simulink model "standModel"  (R2020b)
settings: Solver=VariableStepAuto  StartTime=0.0  StopTime=10.0  RelTol=1e-3
model workspace: external: MAT-File C:\Code\KillerWhaleSim\standParams.mat (data not in the file)
undefined symbols (not defined in the file or in its folder): standParams, X, Y, Z
libraries: sm_lib x713, nesl_utility x1
(part 1 of 11)
settings Model: Creator=roadrunner  LastModifiedBy=roadrunner

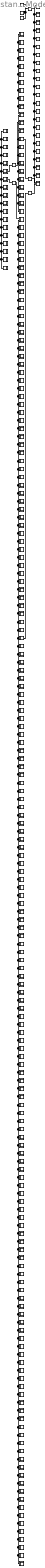
== system standModel ==
  Bracket_16_RIGID : Subsystem
  Bracket_17_RIGID : Subsystem
  Bracket_18_RIGID : Subsystem
  Bracket_19_RIGID : Subsystem
  Bracket_20_RIGID : Subsystem
  Bracket_21_RIGID : Subsystem
  Frame_Part_5_RIGID : Subsystem
  Frame_Part_6_RIGID : Subsystem
  Hinge_10_RIGID : Subsystem
  Hinge_11_RIGID : Subsystem
  Lock_tabs_13_RIGID : Subsystem
  Lock_tabs_15_RIGID : Subsystem
  Lock_tabs_16_RIGID : Subsystem
  Lock_tabs_18_RIGID : Subsystem
  MechanismConfiguration : sm_lib/Utilities/Mechanism Configuration  UniformGravity=Constant  GravityVector=[0 -9.80665 0]  GravityVectorUnits=m/s^2  GravityUnits=m/s^2  LinearizationDelta=0.001  JointModeTransitionNonlinearIterations=2
  Part_132_2_RIGID : Subsystem
  Part_133_2_RIGID : Subsystem
  Part_144_1_RIGID : Subsystem
  Part_145_1_RIGID : Subsystem
  Part_146_1_RIGID : Subsystem
  Part_147_1_RIGID : Subsystem
  Part_148_1_RIGID : Subsystem
  Part_149_1_RIGID : Subsystem
  Part_150_1_RIGID : Subsystem
  Part_151_1_RIGID : Subsystem
  Part_152_1_RIGID : Subsystem
  Part_153_1_RIGID : Subsystem
  Part_154_1_RIGID : Subsystem
  Part_155_1_RIGID : Subsystem
  Part_156_2_RIGID : Subsystem
  Part_157_2_RIGID : Subsystem
  Part_168_1_RIGID : Subsystem
  Part_169_1_RIGID : Subsystem
  Part_170_1_RIGID : Subsystem
  Part_171_1_RIGID : Subsystem
  Part_172_1_RIGID : Subsystem
  Part_173_1_RIGID : Subsystem
  Part_174_1_RIGID : Subsystem
  Part_175_1_RIGID : Subsystem
  Part_176_1_RIGID : Subsystem
  Part_177_1_RIGID : Subsystem
  Part_178_1_RIGID : Subsystem
  Part_179_1_RIGID : Subsystem
  Part_186_1_RIGID : Subsystem
  Part_187_1_RIGID : Subsystem
  Part_188_1_RIGID : Subsystem
  Part_190_1_RIGID : Subsystem
  Part_191_1_RIGID : Subsystem
  Part_192_1_RIGID : Subsystem
  Part_193_1_RIGID : Subsystem
  Part_194_1_RIGID : Subsystem
  Part_195_1_RIGID : Subsystem
  Part_196_1_RIGID : Subsystem
  Part_197_1_RIGID : Subsystem
  Part_198_2_RIGID : Subsystem
  Part_199_2_RIGID : Subsystem
  Part_200_2_RIGID : Subsystem
  Part_204_2_RIGID : Subsystem
  Part_205_2_RIGID : Subsystem
  Part_206_2_RIGID : Subsystem
  Part_213_1_RIGID : Subsystem
  Part_289_1_RIGID : Subsystem
  Part_318_1_RIGID : Subsystem
  Part_319_1_RIGID : Subsystem
  Part_322_1_RIGID : Subsystem
  Part_325_1_RIGID : Subsystem
  Part_328_1_RIGID : Subsystem
  Part_331_1_RIGID : Subsystem
  Part_334_1_RIGID : Subsystem
  Part_337_1_RIGID : Subsystem
  Part_340_1_RIGID : Subsystem
  Part_343_1_RIGID : Subsystem
  Part_346_1_RIGID : Subsystem
  Part_349_1_RIGID : Subsystem
  Part_350_2_RIGID : Subsystem
  Part_351_2_RIGID : Subsystem
  Part_352_2_RIGID : Subsystem
  Part_353_2_RIGID : Subsystem
  Part_355_2_RIGID : Subsystem
  Part_356_2_RIGID : Subsystem
  Part_357_2_RIGID : Subsystem
  Part_358_2_RIGID : Subsystem
  Part_359_2_RIGID : Subsystem
  Part_360_1_RIGID : Subsystem
  Part_361_1_RIGID : Subsystem
  Part_362_1_RIGID : Subsystem
  Part_363_1_RIGID : Subsystem
  Part_364_1_RIGID : Subsystem
  Part_365_1_RIGID : Subsystem
  Part_366_1_RIGID : Subsystem
  Part_367_1_RIGID : Subsystem
  Part_368_1_RIGID : Subsystem
  Part_369_1_RIGID : Subsystem
  Part_370_1_RIGID : Subsystem
  Part_371_1_RIGID : Subsystem
  Part_372_1_RIGID : Subsystem
  Part_373_1_RIGID : Subsystem
  Part_374_1_RIGID : Subsystem
  Part_375_1_RIGID : Subsystem
  Part_380_1_RIGID : Subsystem
  Part_386_1_RIGID : Subsystem
  Part_387_1_RIGID : Subsystem
  Part_393_1_RIGID : Subsystem
  Part_399_1_RIGID : Subsystem
  Part_400_1_RIGID : Subsystem
  Part_406_1_RIGID : Subsystem
  Part_412_1_RIGID : Subsystem
  Part_413_1_RIGID : Subsystem
  Revolute1 : sm_lib/Joints/Revolute Joint  JointMode=Normal  SenseConstraintForce=off  SenseConstraintForceX=off  SenseConstraintForceY=off  SenseConstraintForceZ=off  SenseConstraintTorque=off  SenseConstraintTorqueX=off  SenseConstraintTorqueY=off  SenseConstraintTorqueZ=off  SenseTotalForce=off  SenseTotalForceX=off  SenseTotalForceY=off  SenseTotalForceZ=off  SenseTotalTorque=off  SenseTotalTorqueX=off  SenseTotalTorqueY=off  SenseTotalTorqueZ=off  CompositeWrenchDir=FollowerOnBase  CompositeWrenchFrame=BaseFrame  EquilibriumPosition=0  EquilibriumPositionUnits=deg  SpringStiffness=0  SpringStiffnessUnits=N*m/deg  DampingCoefficient=0  DampingCoefficientUnits=N*m/(deg/s)  TorqueActuationMode=NoTorque  MotionActuationMode=ComputedMotion  SensePosition=off  SenseVelocity=off  SenseAcceleration=off  SenseTorqueForce=off  SenseLowerLimitTorqueForce=off  SenseUpperLimitTorqueForce=off  LowerLimitSpecify=off  LowerLimitBound=-90  LowerLimitBoundUnits=deg  LowerLimitStiffness=1e4  LowerLimitStiffnessUnits=N*m/deg  LowerLimitDamping=10  LowerLimitDampingUnits=N*m/(deg/s)  LowerLimitTransitionRegionWidth=0.1  LowerLimitTransitionRegionWidthUnits=deg  UpperLimitSpecify=off  UpperLimitBound=90  UpperLimitBoundUnits=deg  UpperLimitStiffness=1e4  UpperLimitStiffnessUnits=N*m/deg  UpperLimitDamping=10  UpperLimitDampingUnits=N*m/(deg/s)  UpperLimitTransitionRegionWidth=0.1  UpperLimitTransitionRegionWidthUnits=deg  PositionTargetSpecify=on  PositionTargetPriority=Low  PositionTargetValue=standParams.RevoluteJoint(1).Rz.Pos  PositionTargetValueUnits=deg  VelocityTargetSpecify=off  VelocityTargetPriority=High  VelocityTargetValue=0  VelocityTargetValueUnits=deg/s
  Revolute2 : sm_lib/Joints/Revolute Joint  JointMode=Normal  SenseConstraintForce=off  SenseConstraintForceX=off  SenseConstraintForceY=off  SenseConstraintForceZ=off  SenseConstraintTorque=off  SenseConstraintTorqueX=off  SenseConstraintTorqueY=off  SenseConstraintTorqueZ=off  SenseTotalForce=off  SenseTotalForceX=off  SenseTotalForceY=off  SenseTotalForceZ=off  SenseTotalTorque=off  SenseTotalTorqueX=off  SenseTotalTorqueY=off  SenseTotalTorqueZ=off  CompositeWrenchDir=FollowerOnBase  CompositeWrenchFrame=BaseFrame  EquilibriumPosition=0  EquilibriumPositionUnits=deg  SpringStiffness=0  SpringStiffnessUnits=N*m/deg  DampingCoefficient=0  DampingCoefficientUnits=N*m/(deg/s)  TorqueActuationMode=NoTorque  MotionActuationMode=ComputedMotion  SensePosition=off  SenseVelocity=off  SenseAcceleration=off  SenseTorqueForce=off  SenseLowerLimitTorqueForce=off  SenseUpperLimitTorqueForce=off  LowerLimitSpecify=off  LowerLimitBound=-90  LowerLimitBoundUnits=deg  LowerLimitStiffness=1e4  LowerLimitStiffnessUnits=N*m/deg  LowerLimitDamping=10  LowerLimitDampingUnits=N*m/(deg/s)  LowerLimitTransitionRegionWidth=0.1  LowerLimitTransitionRegionWidthUnits=deg  UpperLimitSpecify=off  UpperLimitBound=90  UpperLimitBoundUnits=deg  UpperLimitStiffness=1e4  UpperLimitStiffnessUnits=N*m/deg  UpperLimitDamping=10  UpperLimitDampingUnits=N*m/(deg/s)  UpperLimitTransitionRegionWidth=0.1  UpperLimitTransitionRegionWidthUnits=deg  PositionTargetSpecify=off  PositionTargetPriority=High  PositionTargetValue=0  PositionTargetValueUnits=deg  VelocityTargetSpecify=off  VelocityTargetPriority=High  VelocityTargetValue=0  VelocityTargetValueUnits=deg/s
  Revolute3 : sm_lib/Joints/Revolute Joint  JointMode=Normal  SenseConstraintForce=off  SenseConstraintForceX=off  SenseConstraintForceY=off  SenseConstraintForceZ=off  SenseConstraintTorque=off  SenseConstraintTorqueX=off  SenseConstraintTorqueY=off  SenseConstraintTorqueZ=off  SenseTotalForce=off  SenseTotalForceX=off  SenseTotalForceY=off  SenseTotalForceZ=off  SenseTotalTorque=off  SenseTotalTorqueX=off  SenseTotalTorqueY=off  SenseTotalTorqueZ=off  CompositeWrenchDir=FollowerOnBase  CompositeWrenchFrame=BaseFrame  EquilibriumPosition=0  EquilibriumPositionUnits=deg  SpringStiffness=0  SpringStiffnessUnits=N*m/deg  DampingCoefficient=0  DampingCoefficientUnits=N*m/(deg/s)  TorqueActuationMode=NoTorque  MotionActuationMode=ComputedMotion  SensePosition=off  SenseVelocity=off  SenseAcceleration=off  SenseTorqueForce=off  SenseLowerLimitTorqueForce=off  SenseUpperLimitTorqueForce=off  LowerLimitSpecify=off  LowerLimitBound=-90  LowerLimitBoundUnits=deg  LowerLimitStiffness=1e4  LowerLimitStiffnessUnits=N*m/deg  LowerLimitDamping=10  LowerLimitDampingUnits=N*m/(deg/s)  LowerLimitTransitionRegionWidth=0.1  LowerLimitTransitionRegionWidthUnits=deg  UpperLimitSpecify=off  UpperLimitBound=90  UpperLimitBoundUnits=deg  UpperLimitStiffness=1e4  UpperLimitStiffnessUnits=N*m/deg  UpperLimitDamping=10  UpperLimitDampingUnits=N*m/(deg/s)  UpperLimitTransitionRegionWidth=0.1  UpperLimitTransitionRegionWidthUnits=deg  PositionTargetSpecify=on  PositionTargetPriority=Low  PositionTargetValue=standParams.RevoluteJoint(2).Rz.Pos  PositionTargetValueUnits=deg  VelocityTargetSpecify=off  VelocityTargetPriority=High  VelocityTargetValue=0  VelocityTargetValueUnits=deg/s
  Revolute4 : sm_lib/Joints/Revolute Joint  JointMode=Normal  SenseConstraintForce=off  SenseConstraintForceX=off  SenseConstraintForceY=off  SenseConstraintForceZ=off  SenseConstraintTorque=off  SenseConstraintTorqueX=off  SenseConstraintTorqueY=off  SenseConstraintTorqueZ=off  SenseTotalForce=off  SenseTotalForceX=off  SenseTotalForceY=off  SenseTotalForceZ=off  SenseTotalTorque=off  SenseTotalTorqueX=off  SenseTotalTorqueY=off  SenseTotalTorqueZ=off  CompositeWrenchDir=FollowerOnBase  CompositeWrenchFrame=BaseFrame  EquilibriumPosition=0  EquilibriumPositionUnits=deg  SpringStiffness=0  SpringStiffnessUnits=N*m/deg  DampingCoefficient=0  DampingCoefficientUnits=N*m/(deg/s)  TorqueActuationMode=NoTorque  MotionActuationMode=ComputedMotion  SensePosition=off  SenseVelocity=off  SenseAcceleration=off  SenseTorqueForce=off  SenseLowerLimitTorqueForce=off  SenseUpperLimitTorqueForce=off  LowerLimitSpecify=off  LowerLimitBound=-90  LowerLimitBoundUnits=deg  LowerLimitStiffness=1e4  LowerLimitStiffnessUnits=N*m/deg  LowerLimitDamping=10  LowerLimitDampingUnits=N*m/(deg/s)  LowerLimitTransitionRegionWidth=0.1  LowerLimitTransitionRegionWidthUnits=deg  UpperLimitSpecify=off  UpperLimitBound=90  UpperLimitBoundUnits=deg  UpperLimitStiffness=1e4  UpperLimitStiffnessUnits=N*m/deg  UpperLimitDamping=10  UpperLimitDampingUnits=N*m/(deg/s)  UpperLimitTransitionRegionWidth=0.1  UpperLimitTransitionRegionWidthUnits=deg  PositionTargetSpecify=on  PositionTargetPriority=Low  PositionTargetValue=standParams.RevoluteJoint(3).Rz.Pos  PositionTargetValueUnits=deg  VelocityTargetSpecify=off  VelocityTargetPriority=High  VelocityTargetValue=0  VelocityTargetValueUnits=deg/s
  Screw_10_3_4_in_10_RIGID : Subsystem
  Screw_10_3_4_in_11_RIGID : Subsystem
  Screw_10_3_4_in_12_RIGID : Subsystem
  Screw_10_3_4_in_13_RIGID : Subsystem
  Screw_10_3_4_in_14_RIGID : Subsystem
  Screw_10_3_4_in_15_RIGID : Subsystem
  Screw_10_3_4_in_16_RIGID : Subsystem
  Screw_10_3_4_in_1_RIGID : Subsystem
  Screw_10_3_4_in_20_RIGID : Subsystem
  Screw_10_3_4_in_21_RIGID : Subsystem
  Screw_10_3_4_in_22_RIGID : Subsystem
  Screw_10_3_4_in_23_RIGID : Subsystem
  Screw_10_3_4_in_24_RIGID : Subsystem
  Screw_10_3_4_in_25_RIGID : Subsystem
  Screw_10_3_4_in_26_RIGID : Subsystem
  Screw_10_3_4_in_27_RIGID : Subsystem
  Screw_10_3_4_in_28_RIGID : Subsystem
  Screw_10_3_4_in_29_RIGID : Subsystem
  Screw_10_3_4_in_30_RIGID : Subsystem
  Screw_10_3_4_in_31_RIGID : Subsystem
  Screw_10_3_4_in_32_RIGID : Subsystem
  Screw_10_3_4_in_33_RIGID : Subsystem
  Screw_10_3_4_in_34_RIGID : Subsystem
  Screw_10_3_4_in_38_RIGID : Subsystem
  Screw_10_3_4_in_5_RIGID : Subsystem
  Screw_10_3_4_in_7_RIGID : Subsystem
  Screw_10_3_4_in_8_RIGID : Subsystem
  Screw_10_3_4_in_9_RIGID : Subsystem
  Screw_8_1_2_in_11_RIGID : Subsystem
  Screw_8_1_2_in_13_RIGID : Subsystem
  Screw_8_1_2_in_14_RIGID : Subsystem
  Screw_8_1_2_in_16_RIGID : Subsystem
  Set_Screw_4_1_4_in_19_RIGID : Subsystem
  Set_Screw_4_1_4_in_20_RIGID : Subsystem
  Set_Screw_4_1_4_in_21_RIGID : Subsystem
  Set_Screw_4_1_4_in_22_RIGID : Subsystem
  Set_Screw_4_1_4_in_23_RIGID : Subsystem
  Set_Screw_4_1_4_in_24_RIGID : Subsystem
  Solver Configuration : nesl_utility/Solver Configuration  PhysicalDomain=network_engine_domain  SubClassName=solver  LeftPortType=input  RightPortType=generic  Tones=[]  Harmonics=[]  SimulateNoise=off  Profile=off  UseLocalSampling=off  EnableSwitchedLinearOptims=on  FrequencyDomain=off  UseCCode=off  RelTol=0.001  AbsTol=1e-06  MinStep=1e-09  ToWorkspace=off  RevertToSquareIcSolve=off  NumHomotopyIterations=100  PhasorMode=off  PhasorModeNumHarmonics=1  DoDC=off  ResidualTolerance=1e-09  UseLocalSolver=off  LocalSolverChoice=NE_BACKWARD_EULER_ADVANCER  LocalSolverSampleTime=0.001  DoFixedCost=off  MaxNonlinIter=3  MaxModeIter=2  ComputeImpulses=off  ImpulseIterations=2  LinearAlgebra=auto  EquationFormulation=NE_TIME_EF  DelaysMemoryBudget=1024  AutomaticFiltering=on  FilteringTimeConstant=0.001  PartitionStorageMethod=AS_NEEDED  PartitionMemoryBudget=1024  PartitionMethod=ROBUST
  Spacer_19_RIGID : Subsystem
  Spacer_21_RIGID : Subsystem
  Spacer_22_RIGID : Subsystem
  Spacer_24_RIGID : Subsystem
  Spring_Pin_1_8_in_OD_1_4_in_L_100_RIGID : Subsystem
  Spring_Pin_1_8_in_OD_1_4_in_L_101_RIGID : Subsystem
  Spring_Pin_1_8_in_OD_1_4_in_L_12_RIGID : Subsystem
  Spring_Pin_1_8_in_OD_1_4_in_L_55_RIGID : Subsystem
  Spring_Pin_1_8_in_OD_1_4_in_L_56_RIGID : Subsystem
  Spring_Pin_1_8_in_OD_1_4_in_L_57_RIGID : Subsystem
  Spring_Pin_1_8_in_OD_1_4_in_L_58_RIGID : Subsystem
  Spring_Pin_1_8_in_OD_1_4_in_L_59_RIGID : Subsystem
  Spring_Pin_1_8_in_OD_1_4_in_L_60_RIGID : Subsystem
  Spring_Pin_1_8_in_OD_1_4_in_L_61_RIGID : Subsystem
  Spring_Pin_1_8_in_OD_1_4_in_L_62_RIGID : Subsystem
  Spring_Pin_1_8_in_OD_1_4_in_L_63_RIGID : Subsystem
  Spring_Pin_1_8_in_OD_1_4_in_L_64_RIGID : Subsystem
  Spring_Pin_1_8_in_OD_1_4_in_L_65_RIGID : Subsystem
  Spring_Pin_1_8_in_OD_1_4_in_L_66_RIGID : Subsystem
  Spring_Pin_1_8_in_OD_1_4_in_L_67_RIGID : Subsystem
  Spring_Pin_1_8_in_OD_1_4_in_L_68_RIGID : Subsystem
  Spring_Pin_1_8_in_OD_1_4_in_L_69_RIGID : Subsystem
  Spring_Pin_1_8_in_OD_1_4_in_L_70_RIGID : Subsystem
  Spring_Pin_1_8_in_OD_1_4_in_L_71_RIGID : Subsystem
  Spring_Pin_1_8_in_OD_1_4_in_L_72_RIGID : Subsystem
  Spring_Pin_1_8_in_OD_1_4_in_L_73_RIGID : Subsystem
  Spring_Pin_1_8_in_OD_1_4_in_L_74_RIGID : Subsystem
  Spring_Pin_1_8_in_OD_1_4_in_L_75_RIGID : Subsystem
  Spring_Pin_1_8_in_OD_1_4_in_L_76_RIGID : Subsystem
  Spring_Pin_1_8_in_OD_1_4_in_L_77_RIGID : Subsystem
  Spring_Pin_1_8_in_OD_1_4_in_L_78_RIGID : Subsystem
  Spring_Pin_1_8_in_OD_1_4_in_L_79_RIGID : Subsystem
  Spring_Pin_1_8_in_OD_1_4_in_L_80_RIGID : Subsystem
  Spring_Pin_1_8_in_OD_1_4_in_L_81_RIGID : Subsystem
  Spring_Pin_1_8_in_OD_1_4_in_L_82_RIGID : Subsystem
  Spring_Pin_1_8_in_OD_1_4_in_L_83_RIGID : Subsystem
  Spring_Pin_1_8_in_OD_1_4_in_L_84_RIGID : Subsystem
  Spring_Pin_1_8_in_OD_1_4_in_L_85_RIGID : Subsystem
  Spring_Pin_1_8_in_OD_1_4_in_L_86_RIGID : Subsystem
  Spring_Pin_1_8_in_OD_1_4_in_L_87_RIGID : Subsystem
  Spring_Pin_1_8_in_OD_1_4_in_L_88_RIGID : Subsystem
  Spring_Pin_1_8_in_OD_1_4_in_L_89_RIGID : Subsystem
  Spring_Pin_1_8_in_OD_1_4_in_L_90_RIGID : Subsystem
  Spring_Pin_1_8_in_OD_1_4_in_L_91_RIGID : Subsystem
  Spring_Pin_1_8_in_OD_1_4_in_L_92_RIGID : Subsystem
  Spring_Pin_1_8_in_OD_1_4_in_L_93_RIGID : Subsystem
  Spring_Pin_1_8_in_OD_1_4_in_L_94_RIGID : Subsystem
  Spring_Pin_1_8_in_OD_1_4_in_L_96_RIGID : Subsystem
  Spring_Pin_1_8_in_OD_1_4_in_L_97_RIGID : Subsystem
  Spring_Pin_1_8_in_OD_1_4_in_L_98_RIGID : Subsystem
  Spring_Pin_1_8_in_OD_1_4_in_L_99_RIGID : Subsystem
  Standoff_4_RIGID : Subsystem
  Standoff_5_RIGID : Subsystem
  Transform : sm_lib/Frames and Transforms/Rigid Transform  TranslationMethod=Cartesian  TranslationStandardOffset=0  TranslationLengthUnit=in  TranslationStandardAxis=+Z  TranslationCartesianOffset=standParams.RigidTransform(243).translation  TranslationROffset=0  TranslationROffsetUnits=m  TranslationZOffset=0  TranslationZOffsetUnits=m  TranslationThetaOffset=0  TranslationThetaOffsetUnits=deg  RotationMethod=ArbitraryAxis  RotationAngleUnits=rad  RotationStandardAxis=+Z  RotationAngle=standParams.RigidTransform(243).angle  RotationArbitraryAxis=standParams.RigidTransform(243).axis  FollAlignAxisA=+X  BaseAlignAxisA=+Y  FollAlignAxisB=+Y  BaseAlignAxisB=+Z  RotationSequenceAxes=FollowerAxes  RotationSequence=XYX  RotationSequenceAngles=[0 0 0]  RotationSequenceAnglesUnits=deg  RotationMatrix=[1 0 0; 0 1 0; 0 0 1]
  Washer_10_10_RIGID : Subsystem
  Washer_10_11_RIGID : Subsystem
  Washer_10_12_RIGID : Subsystem
  Washer_10_13_RIGID : Subsystem
  Washer_10_14_RIGID : Subsystem
  Washer_10_15_RIGID : Subsystem
  Washer_10_16_RIGID : Subsystem
  Washer_10_17_RIGID : Subsystem
  Washer_10_18_RIGID : Subsystem
  Washer_10_20_RIGID : Subsystem
  Washer_10_21_RIGID : Subsystem
  Washer_10_22_RIGID : Subsystem
  Washer_10_23_RIGID : Subsystem
  Washer_10_24_RIGID : Subsystem
  Washer_10_25_RIGID : Subsystem
  Washer_10_26_RIGID : Subsystem
  Washer_10_27_RIGID : Subsystem
  Washer_10_28_RIGID : Subsystem
  Washer_10_29_RIGID : Subsystem
  Washer_10_30_RIGID : Subsystem
  Washer_10_31_RIGID : Subsystem
  Washer_10_7_RIGID : Subsystem
  Washer_10_8_RIGID : Subsystem
  Washer_10_9_RIGID : Subsystem
  Washer_8_13_RIGID : Subsystem
  Washer_8_15_RIGID : Subsystem
  Washer_8_16_RIGID : Subsystem
  Washer_8_18_RIGID : Subsystem
  World : sm_lib/Frames and Transforms/World Frame
  forward_torso_l_2_RIGID : Subsystem
  forward_torso_l_3_RIGID : Subsystem
  forward_torso_l_4_RIGID : Subsystem
  forward_torso_l_5_RIGID : Subsystem
  forward_torso_l_6_RIGID : Subsystem
  nut_1_RIGID : Subsystem
  connections:
  Transform/LConn1 -- MechanismConfiguration/RConn1 -- Solver Configuration/RConn1 -- World/RConn1
  Frame_Part_6_RIGID/LConn1 -- Frame_Part_5_RIGID/LConn1 -- Washer_8_16_RIGID/LConn1 -- Washer_8_18_RIGID/LConn1 -- Washer_8_15_RIGID/LConn1 -- Washer_8_13_RIGID/LConn1 -- Spacer_24_RIGID/LConn1 -- Spacer_21_RIGID/LConn1 -- Spacer_22_RIGID/LConn1 -- Spacer_19_RIGID/LConn1 -- Screw_8_1_2_in_16_RIGID/LConn1 -- Screw_8_1_2_in_14_RIGID/LConn1 -- Screw_8_1_2_in_13_RIGID/LConn1 -- Screw_8_1_2_in_11_RIGID/LConn1 -- Lock_tabs_18_RIGID/LConn1 -- Lock_tabs_16_RIGID/LConn1 -- Lock_tabs_15_RIGID/LConn1 -- Lock_tabs_13_RIGID/LConn1
  Revolute4/LConn1 -- Standoff_5_RIGID/RConn1
  Part_356_2_RIGID/LConn2 -- Revolute4/RConn1
  Revolute2/LConn1 -- Spacer_21_RIGID/RConn1
  Part_289_1_RIGID/LConn2 -- Revolute2/RConn1
  Bracket_18_RIGID/LConn2 -- Part_289_1_RIGID/LConn1
  Part_359_2_RIGID/LConn1 -- Transform/RConn1
  Bracket_21_RIGID/LConn1 -- Spring_Pin_1_8_in_OD_1_4_in_L_63_RIGID/LConn1 -- Spring_Pin_1_8_in_OD_1_4_in_L_70_RIGID/LConn1 -- Spring_Pin_1_8_in_OD_1_4_in_L_62_RIGID/LConn1 -- Spring_Pin_1_8_in_OD_1_4_in_L_61_RIGID/LConn1 -- Set_Screw_4_1_4_in_24_RIGID/LConn1 -- Set_Screw_4_1_4_in_21_RIGID/LConn1 -- Hinge_11_RIGID/LConn1 -- Bracket_18_RIGID/LConn1 -- Spring_Pin_1_8_in_OD_1_4_in_L_71_RIGID/LConn1 -- Spring_Pin_1_8_in_OD_1_4_in_L_72_RIGID/LConn1
  Part_289_1_RIGID/LConn3 -- Part_213_1_RIGID/LConn1 -- Washer_10_18_RIGID/LConn1 -- Washer_10_20_RIGID/LConn1 -- Washer_10_21_RIGID/LConn1 -- Standoff_5_RIGID/LConn1 -- Washer_10_17_RIGID/LConn1 -- Standoff_4_RIGID/LConn1 -- Screw_10_3_4_in_24_RIGID/LConn1 -- Screw_10_3_4_in_23_RIGID/LConn1 -- Screw_10_3_4_in_21_RIGID/LConn1 -- Screw_10_3_4_in_20_RIGID/LConn1
  Bracket_17_RIGID/LConn1 -- Part_318_1_RIGID/LConn2 -- Part_371_1_RIGID/LConn1 -- Part_370_1_RIGID/LConn1 -- Part_369_1_RIGID/LConn1 -- Part_368_1_RIGID/LConn1 -- Part_367_1_RIGID/LConn1 -- Part_366_1_RIGID/LConn1 -- Part_365_1_RIGID/LConn1 -- Part_364_1_RIGID/LConn1 -- Part_363_1_RIGID/LConn1 -- Part_362_1_RIGID/LConn1 -- Part_361_1_RIGID/LConn1 -- Part_360_1_RIGID/LConn1 -- Part_349_1_RIGID/LConn1 -- Part_346_1_RIGID/LConn1 -- Part_343_1_RIGID/LConn1 -- Part_340_1_RIGID/LConn1 -- Part_337_1_RIGID/LConn1 -- Part_334_1_RIGID/LConn1 -- Part_331_1_RIGID/LConn1 -- Part_328_1_RIGID/LConn1 -- Part_325_1_RIGID/LConn1 -- Part_322_1_RIGID/LConn1 -- Part_319_1_RIGID/LConn1 -- Part_197_1_RIGID/LConn1 -- Part_196_1_RIGID/LConn1 -- Part_195_1_RIGID/LConn1 -- Part_194_1_RIGID/LConn1 -- Part_193_1_RIGID/LConn1 -- Part_192_1_RIGID/LConn1 -- Part_191_1_RIGID/LConn1 -- Part_190_1_RIGID/LConn1 -- Part_188_1_RIGID/LConn1 -- Part_187_1_RIGID/LConn1 -- Part_186_1_RIGID/LConn1 -- Part_179_1_RIGID/LConn1 -- Part_178_1_RIGID/LConn1 -- Part_177_1_RIGID/LConn1 -- Part_176_1_RIGID/LConn1 -- Part_175_1_RIGID/LConn1 -- Part_174_1_RIGID/LConn1 -- Part_173_1_RIGID/LConn1 -- Part_172_1_RIGID/LConn1 -- Part_171_1_RIGID/LConn1 -- Part_170_1_RIGID/LConn1 -- Part_169_1_RIGID/LConn1 -- Part_168_1_RIGID/LConn1 -- Part_155_1_RIGID/LConn1 -- Part_154_1_RIGID/LConn1 -- Part_153_1_RIGID/LConn1 -- Part_152_1_RIGID/LConn1 -- Part_151_1_RIGID/LConn1 -- Part_150_1_RIGID/LConn1 -- Part_149_1_RIGID/LConn1 -- Part_148_1_RIGID/LConn1 -- Part_147_1_RIGID/LConn1 -- Part_146_1_RIGID/LConn1 -- Part_145_1_RIGID/LConn1 -- Part_144_1_RIGID/LConn1 -- Hinge_10_RIGID/LConn1 -- Bracket_20_RIGID/LConn1 -- Bracket_19_RIGID/LConn1 -- Bracket_16_RIGID/LConn1 -- Part_372_1_RIGID/LConn1 -- Part_373_1_RIGID/LConn1 -- Part_374_1_RIGID/LConn1 -- Part_375_1_RIGID/LConn1 -- Part_380_1_RIGID/LConn1 -- Part_386_1_RIGID/LConn1 -- Part_387_1_RIGID/LConn1 -- Part_393_1_RIGID/LConn1 -- Part_399_1_RIGID/LConn1 -- Part_400_1_RIGID/LConn1 -- Part_406_1_RIGID/LConn1 -- Part_412_1_RIGID/LConn1 -- Part_413_1_RIGID/LConn1 -- Screw_10_3_4_in_10_RIGID/LConn1 -- Screw_10_3_4_in_11_RIGID/LConn1 -- Screw_10_3_4_in_12_RIGID/LConn1 -- Screw_10_3_4_in_13_RIGID/LConn1 -- Screw_10_3_4_in_14_RIGID/LConn1 -- Screw_10_3_4_in_15_RIGID/LConn1 -- Screw_10_3_4_in_16_RIGID/LConn1 -- Screw_10_3_4_in_25_RIGID/LConn1 -- Screw_10_3_4_in_26_RIGID/LConn1 -- Screw_10_3_4_in_27_RIGID/LConn1 -- Screw_10_3_4_in_28_RIGID/LConn1 -- Screw_10_3_4_in_29_RIGID/LConn1 -- Screw_10_3_4_in_30_RIGID/LConn1 -- Screw_10_3_4_in_31_RIGID/LConn1 -- Screw_10_3_4_in_32_RIGID/LConn1 -- Screw_10_3_4_in_33_RIGID/LConn1 -- Screw_10_3_4_in_34_RIGID/LConn1 -- Screw_10_3_4_in_7_RIGID/LConn1 -- Screw_10_3_4_in_8_RIGID/LConn1 -- Screw_10_3_4_in_9_RIGID/LConn1 -- Set_Screw_4_1_4_in_19_RIGID/LConn1 -- Set_Screw_4_1_4_in_20_RIGID/LConn1 -- Set_Screw_4_1_4_in_22_RIGID/LConn1 -- Set_Screw_4_1_4_in_23_RIGID/LConn1 -- Spring_Pin_1_8_in_OD_1_4_in_L_100_RIGID/LConn1 -- Spring_Pin_1_8_in_OD_1_4_in_L_101_RIGID/LConn1 -- Spring_Pin_1_8_in_OD_1_4_in_L_12_RIGID/LConn1 -- Spring_Pin_1_8_in_OD_1_4_in_L_55_RIGID/LConn1 -- Spring_Pin_1_8_in_OD_1_4_in_L_56_RIGID/LConn1 -- Spring_Pin_1_8_in_OD_1_4_in_L_57_RIGID/LConn1 -- Spring_Pin_1_8_in_OD_1_4_in_L_58_RIGID/LConn1 -- Spring_Pin_1_8_in_OD_1_4_in_L_59_RIGID/LConn1 -- Spring_Pin_1_8_in_OD_1_4_in_L_60_RIGID/LConn1 -- Spring_Pin_1_8_in_OD_1_4_in_L_64_RIGID/LConn1 -- Spring_Pin_1_8_in_OD_1_4_in_L_65_RIGID/LConn1 -- Spring_Pin_1_8_in_OD_1_4_in_L_66_RIGID/LConn1 -- Spring_Pin_1_8_in_OD_1_4_in_L_67_RIGID/LConn1 -- Spring_Pin_1_8_in_OD_1_4_in_L_68_RIGID/LConn1 -- Spring_Pin_1_8_in_OD_1_4_in_L_69_RIGID/LConn1 -- Spring_Pin_1_8_in_OD_1_4_in_L_73_RIGID/LConn1 -- Spring_Pin_1_8_in_OD_1_4_in_L_74_RIGID/LConn1 -- Spring_Pin_1_8_in_OD_1_4_in_L_75_RIGID/LConn1 -- Spring_Pin_1_8_in_OD_1_4_in_L_76_RIGID/LConn1 -- Spring_Pin_1_8_in_OD_1_4_in_L_77_RIGID/LConn1 -- Spring_Pin_1_8_in_OD_1_4_in_L_78_RIGID/LConn1 -- Spring_Pin_1_8_in_OD_1_4_in_L_79_RIGID/LConn1 -- Spring_Pin_1_8_in_OD_1_4_in_L_80_RIGID/LConn1 -- Spring_Pin_1_8_in_OD_1_4_in_L_81_RIGID/LConn1 -- Spring_Pin_1_8_in_OD_1_4_in_L_82_RIGID/LConn1 -- Spring_Pin_1_8_in_OD_1_4_in_L_83_RIGID/LConn1 -- Spring_Pin_1_8_in_OD_1_4_in_L_84_RIGID/LConn1 -- Spring_Pin_1_8_in_OD_1_4_in_L_85_RIGID/LConn1 -- Spring_Pin_1_8_in_OD_1_4_in_L_86_RIGID/LConn1 -- Spring_Pin_1_8_in_OD_1_4_in_L_87_RIGID/LConn1 -- Spring_Pin_1_8_in_OD_1_4_in_L_88_RIGID/LConn1 -- Spring_Pin_1_8_in_OD_1_4_in_L_89_RIGID/LConn1 -- Spring_Pin_1_8_in_OD_1_4_in_L_90_RIGID/LConn1 -- Spring_Pin_1_8_in_OD_1_4_in_L_91_RIGID/LConn1 -- Spring_Pin_1_8_in_OD_1_4_in_L_92_RIGID/LConn1 -- Spring_Pin_1_8_in_OD_1_4_in_L_93_RIGID/LConn1 -- Spring_Pin_1_8_in_OD_1_4_in_L_94_RIGID/LConn1 -- Spring_Pin_1_8_in_OD_1_4_in_L_96_RIGID/LConn1 -- Spring_Pin_1_8_in_OD_1_4_in_L_97_RIGID/LConn1 -- Spring_Pin_1_8_in_OD_1_4_in_L_98_RIGID/LConn1 -- Spring_Pin_1_8_in_OD_1_4_in_L_99_RIGID/LConn1 -- Washer_10_10_RIGID/LConn1 -- Washer_10_11_RIGID/LConn1 -- Washer_10_12_RIGID/LConn1 -- Washer_10_13_RIGID/LConn1 -- Washer_10_14_RIGID/LConn1 -- Washer_10_15_RIGID/LConn1 -- Washer_10_16_RIGID/LConn1 -- Washer_10_22_RIGID/LConn1 -- Washer_10_23_RIGID/LConn1 -- Washer_10_24_RIGID/LConn1 -- Washer_10_25_RIGID/LConn1 -- Washer_10_26_RIGID/LConn1 -- Washer_10_27_RIGID/LConn1 -- Washer_10_28_RIGID/LConn1 -- Washer_10_29_RIGID/LConn1 -- Washer_10_30_RIGID/LConn1 -- Washer_10_31_RIGID/LConn1 -- Washer_10_7_RIGID/LConn1 -- Washer_10_8_RIGID/LConn1 -- Washer_10_9_RIGID/LConn1 -- forward_torso_l_2_RIGID/LConn1 -- forward_torso_l_3_RIGID/LConn1 -- forward_torso_l_4_RIGID/LConn1 -- forward_torso_l_5_RIGID/LConn1 -- forward_torso_l_6_RIGID/LConn1 -- nut_1_RIGID/LConn1
  Part_133_2_RIGID/LConn1 -- Part_352_2_RIGID/LConn1 -- Part_359_2_RIGID/LConn2 -- Part_351_2_RIGID/LConn1 -- Part_350_2_RIGID/LConn1 -- Part_206_2_RIGID/LConn1 -- Part_205_2_RIGID/LConn1 -- Part_204_2_RIGID/LConn1 -- Part_200_2_RIGID/LConn1 -- Part_199_2_RIGID/LConn1 -- Part_198_2_RIGID/LConn1 -- Part_157_2_RIGID/LConn1 -- Part_156_2_RIGID/LConn1 -- Part_132_2_RIGID/LConn1 -- Part_353_2_RIGID/LConn1 -- Part_356_2_RIGID/LConn1 -- Part_355_2_RIGID/LConn1 -- Part_357_2_RIGID/LConn1 -- Part_358_2_RIGID/LConn1 -- Screw_10_3_4_in_1_RIGID/LConn1 -- Screw_10_3_4_in_22_RIGID/LConn1 -- Screw_10_3_4_in_38_RIGID/LConn1 -- Screw_10_3_4_in_5_RIGID/LConn1
  Part_150_1_RIGID/RConn1 -- Revolute1/LConn1
  Part_356_2_RIGID/LConn3 -- Revolute1/RConn1
  Revolute3/LConn1 -- Spacer_22_RIGID/RConn1
  Part_318_1_RIGID/LConn1 -- Revolute3/RConn1

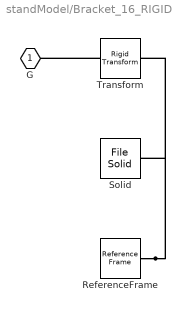
== system standModel/Bracket_16_RIGID ==
  ReferenceFrame : sm_lib/Frames and Transforms/Reference Frame
  Solid : sm_lib/Body Elements/File Solid  ExtGeomFileName=Bracket1.step  UnitType=FromFile  ExtGeomFileUnits=m  StepReaderType=HEX  ExportConvexHullGeometry=off  InertiaType=Custom  Mass=standParams.Solid(64).mass  MassUnits=lbm  CenterOfMass=standParams.Solid(64).CoM  CenterOfMassUnits=in  MomentsOfInertia=standParams.Solid(64).MoI  MomentsOfInertiaUnits=lbm*in^2  ProductsOfInertia=standParams.Solid(64).PoI  ProductsOfInertiaUnits=lbm*in^2  BasedOnType=DensityFromFile  Density=1000  DensityUnits=kg/m^3  DoExposeReferenceFrame=on  SerializedFrames=<Frames/>  GraphicType=FromGeometry  MarkerShape=Sphere  MarkerSize=10  GraphicVisPropType=SimpleVisualProperties  GraphicDiffuseColor=standParams.Solid(64).color  GraphicSpecularColor=[0.5 0.5 0.5 1.0]  GraphicAmbientColor=[0.15 0.15 0.15 1.0]  GraphicEmissiveColor=[0.0 0.0 0.0 1.0]  GraphicShininess=75  GraphicOpacity=standParams.Solid(64).opacity
  Transform : sm_lib/Frames and Transforms/Rigid Transform  TranslationMethod=Cartesian  TranslationStandardOffset=0  TranslationLengthUnit=in  TranslationStandardAxis=+Z  TranslationCartesianOffset=standParams.RigidTransform(88).translation  TranslationROffset=0  TranslationROffsetUnits=m  TranslationZOffset=0  TranslationZOffsetUnits=m  TranslationThetaOffset=0  TranslationThetaOffsetUnits=deg  RotationMethod=ArbitraryAxis  RotationAngleUnits=rad  RotationStandardAxis=+Z  RotationAngle=standParams.RigidTransform(88).angle  RotationArbitraryAxis=standParams.RigidTransform(88).axis  FollAlignAxisA=+X  BaseAlignAxisA=+Y  FollAlignAxisB=+Y  BaseAlignAxisB=+Z  RotationSequenceAxes=FollowerAxes  RotationSequence=XYX  RotationSequenceAngles=[0 0 0]  RotationSequenceAnglesUnits=deg  RotationMatrix=[1 0 0; 0 1 0; 0 0 1]
  G : PMIOPort  Side=Left
  connections:
  Solid/RConn1 -- ReferenceFrame/RConn1 -- Transform/RConn1
  Transform/LConn1 -- G/RConn1

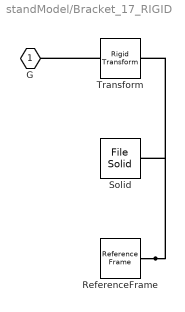
== system standModel/Bracket_17_RIGID ==
  ReferenceFrame : sm_lib/Frames and Transforms/Reference Frame
  Solid : sm_lib/Body Elements/File Solid  ExtGeomFileName=Bracket2.step  UnitType=FromFile  ExtGeomFileUnits=m  StepReaderType=HEX  ExportConvexHullGeometry=off  InertiaType=Custom  Mass=standParams.Solid(37).mass  MassUnits=lbm  CenterOfMass=standParams.Solid(37).CoM  CenterOfMassUnits=in  MomentsOfInertia=standParams.Solid(37).MoI  MomentsOfInertiaUnits=lbm*in^2  ProductsOfInertia=standParams.Solid(37).PoI  ProductsOfInertiaUnits=lbm*in^2  BasedOnType=DensityFromFile  Density=1000  DensityUnits=kg/m^3  DoExposeReferenceFrame=on  SerializedFrames=<Frames/>  GraphicType=FromGeometry  MarkerShape=Sphere  MarkerSize=10  GraphicVisPropType=SimpleVisualProperties  GraphicDiffuseColor=standParams.Solid(37).color  GraphicSpecularColor=[0.5 0.5 0.5 1.0]  GraphicAmbientColor=[0.15 0.15 0.15 1.0]  GraphicEmissiveColor=[0.0 0.0 0.0 1.0]  GraphicShininess=75  GraphicOpacity=standParams.Solid(37).opacity
  Transform : sm_lib/Frames and Transforms/Rigid Transform  TranslationMethod=Cartesian  TranslationStandardOffset=0  TranslationLengthUnit=in  TranslationStandardAxis=+Z  TranslationCartesianOffset=standParams.RigidTransform(67).translation  TranslationROffset=0  TranslationROffsetUnits=m  TranslationZOffset=0  TranslationZOffsetUnits=m  TranslationThetaOffset=0  TranslationThetaOffsetUnits=deg  RotationMethod=ArbitraryAxis  RotationAngleUnits=rad  RotationStandardAxis=+Z  RotationAngle=standParams.RigidTransform(67).angle  RotationArbitraryAxis=standParams.RigidTransform(67).axis  FollAlignAxisA=+X  BaseAlignAxisA=+Y  FollAlignAxisB=+Y  BaseAlignAxisB=+Z  RotationSequenceAxes=FollowerAxes  RotationSequence=XYX  RotationSequenceAngles=[0 0 0]  RotationSequenceAnglesUnits=deg  RotationMatrix=[1 0 0; 0 1 0; 0 0 1]
  G : PMIOPort  Side=Left
  connections:
  Solid/RConn1 -- ReferenceFrame/RConn1 -- Transform/RConn1
  Transform/LConn1 -- G/RConn1

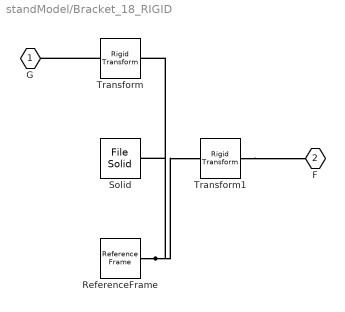
== system standModel/Bracket_18_RIGID ==
  ReferenceFrame : sm_lib/Frames and Transforms/Reference Frame
  Solid : sm_lib/Body Elements/File Solid  ExtGeomFileName=Bracket3.step  UnitType=FromFile  ExtGeomFileUnits=m  StepReaderType=HEX  ExportConvexHullGeometry=off  InertiaType=Custom  Mass=standParams.Solid(168).mass  MassUnits=lbm  CenterOfMass=standParams.Solid(168).CoM  CenterOfMassUnits=in  MomentsOfInertia=standParams.Solid(168).MoI  MomentsOfInertiaUnits=lbm*in^2  ProductsOfInertia=standParams.Solid(168).PoI  ProductsOfInertiaUnits=lbm*in^2  BasedOnType=DensityFromFile  Density=1000  DensityUnits=kg/m^3  DoExposeReferenceFrame=on  SerializedFrames=<Frames/>  GraphicType=FromGeometry  MarkerShape=Sphere  MarkerSize=10  GraphicVisPropType=SimpleVisualProperties  GraphicDiffuseColor=standParams.Solid(168).color  GraphicSpecularColor=[0.5 0.5 0.5 1.0]  GraphicAmbientColor=[0.15 0.15 0.15 1.0]  GraphicEmissiveColor=[0.0 0.0 0.0 1.0]  GraphicShininess=75  GraphicOpacity=standParams.Solid(168).opacity
  Transform : sm_lib/Frames and Transforms/Rigid Transform  TranslationMethod=Cartesian  TranslationStandardOffset=0  TranslationLengthUnit=in  TranslationStandardAxis=+Z  TranslationCartesianOffset=standParams.RigidTransform(28).translation  TranslationROffset=0  TranslationROffsetUnits=m  TranslationZOffset=0  TranslationZOffsetUnits=m  TranslationThetaOffset=0  TranslationThetaOffsetUnits=deg  RotationMethod=ArbitraryAxis  RotationAngleUnits=rad  RotationStandardAxis=+Z  RotationAngle=standParams.RigidTransform(28).angle  RotationArbitraryAxis=standParams.RigidTransform(28).axis  FollAlignAxisA=+X  BaseAlignAxisA=+Y  FollAlignAxisB=+Y  BaseAlignAxisB=+Z  RotationSequenceAxes=FollowerAxes  RotationSequence=XYX  RotationSequenceAngles=[0 0 0]  RotationSequenceAnglesUnits=deg  RotationMatrix=[1 0 0; 0 1 0; 0 0 1]
  Transform1 : sm_lib/Frames and Transforms/Rigid Transform  TranslationMethod=Cartesian  TranslationStandardOffset=0  TranslationLengthUnit=in  TranslationStandardAxis=+Z  TranslationCartesianOffset=standParams.RigidTransform(241).translation  TranslationROffset=0  TranslationROffsetUnits=m  TranslationZOffset=0  TranslationZOffsetUnits=m  TranslationThetaOffset=0  TranslationThetaOffsetUnits=deg  RotationMethod=ArbitraryAxis  RotationAngleUnits=rad  RotationStandardAxis=+Z  RotationAngle=standParams.RigidTransform(241).angle  RotationArbitraryAxis=standParams.RigidTransform(241).axis  FollAlignAxisA=+X  BaseAlignAxisA=+Y  FollAlignAxisB=+Y  BaseAlignAxisB=+Z  RotationSequenceAxes=FollowerAxes  RotationSequence=XYX  RotationSequenceAngles=[0 0 0]  RotationSequenceAnglesUnits=deg  RotationMatrix=[1 0 0; 0 1 0; 0 0 1]
  G : PMIOPort  Side=Left
  F : PMIOPort  Port=2  Side=Left
  connections:
  Solid/RConn1 -- ReferenceFrame/RConn1 -- Transform/RConn1 -- Transform1/LConn1
  Transform/LConn1 -- G/RConn1
  Transform1/RConn1 -- F/RConn1

== system standModel/Bracket_19_RIGID ==
  ReferenceFrame : sm_lib/Frames and Transforms/Reference Frame
  Solid : sm_lib/Body Elements/File Solid  ExtGeomFileName=Bracket4.step  UnitType=FromFile  ExtGeomFileUnits=m  StepReaderType=HEX  ExportConvexHullGeometry=off  InertiaType=Custom  Mass=standParams.Solid(13).mass  MassUnits=lbm  CenterOfMass=standParams.Solid(13).CoM  CenterOfMassUnits=in  MomentsOfInertia=standParams.Solid(13).MoI  MomentsOfInertiaUnits=lbm*in^2  ProductsOfInertia=standParams.Solid(13).PoI  ProductsOfInertiaUnits=lbm*in^2  BasedOnType=DensityFromFile  Density=1000  DensityUnits=kg/m^3  DoExposeReferenceFrame=on  SerializedFrames=<Frames/>  GraphicType=FromGeometry  MarkerShape=Sphere  MarkerSize=10  GraphicVisPropType=SimpleVisualProperties  GraphicDiffuseColor=standParams.Solid(13).color  GraphicSpecularColor=[0.5 0.5 0.5 1.0]  GraphicAmbientColor=[0.15 0.15 0.15 1.0]  GraphicEmissiveColor=[0.0 0.0 0.0 1.0]  GraphicShininess=75  GraphicOpacity=standParams.Solid(13).opacity
  Transform : sm_lib/Frames and Transforms/Rigid Transform  TranslationMethod=Cartesian  TranslationStandardOffset=0  TranslationLengthUnit=in  TranslationStandardAxis=+Z  TranslationCartesianOffset=standParams.RigidTransform(52).translation  TranslationROffset=0  TranslationROffsetUnits=m  TranslationZOffset=0  TranslationZOffsetUnits=m  TranslationThetaOffset=0  TranslationThetaOffsetUnits=deg  RotationMethod=ArbitraryAxis  RotationAngleUnits=rad  RotationStandardAxis=+Z  RotationAngle=standParams.RigidTransform(52).angle  RotationArbitraryAxis=standParams.RigidTransform(52).axis  FollAlignAxisA=+X  BaseAlignAxisA=+Y  FollAlignAxisB=+Y  BaseAlignAxisB=+Z  RotationSequenceAxes=FollowerAxes  RotationSequence=XYX  RotationSequenceAngles=[0 0 0]  RotationSequenceAnglesUnits=deg  RotationMatrix=[1 0 0; 0 1 0; 0 0 1]
  G : PMIOPort  Side=Left
  connections:
  Solid/RConn1 -- ReferenceFrame/RConn1 -- Transform/RConn1
  Transform/LConn1 -- G/RConn1

== system standModel/Bracket_20_RIGID ==
  ReferenceFrame : sm_lib/Frames and Transforms/Reference Frame
  Solid : sm_lib/Body Elements/File Solid  ExtGeomFileName=Bracket5.step  UnitType=FromFile  ExtGeomFileUnits=m  StepReaderType=HEX  ExportConvexHullGeometry=off  InertiaType=Custom  Mass=standParams.Solid(212).mass  MassUnits=lbm  CenterOfMass=standParams.Solid(212).CoM  CenterOfMassUnits=in  MomentsOfInertia=standParams.Solid(212).MoI  MomentsOfInertiaUnits=lbm*in^2  ProductsOfInertia=standParams.Solid(212).PoI  ProductsOfInertiaUnits=lbm*in^2  BasedOnType=DensityFromFile  Density=1000  DensityUnits=kg/m^3  DoExposeReferenceFrame=on  SerializedFrames=<Frames/>  GraphicType=FromGeometry  MarkerShape=Sphere  MarkerSize=10  GraphicVisPropType=SimpleVisualProperties  GraphicDiffuseColor=standParams.Solid(212).color  GraphicSpecularColor=[0.5 0.5 0.5 1.0]  GraphicAmbientColor=[0.15 0.15 0.15 1.0]  GraphicEmissiveColor=[0.0 0.0 0.0 1.0]  GraphicShininess=75  GraphicOpacity=standParams.Solid(212).opacity
  Transform : sm_lib/Frames and Transforms/Rigid Transform  TranslationMethod=Cartesian  TranslationStandardOffset=0  TranslationLengthUnit=in  TranslationStandardAxis=+Z  TranslationCartesianOffset=standParams.RigidTransform(193).translation  TranslationROffset=0  TranslationROffsetUnits=m  TranslationZOffset=0  TranslationZOffsetUnits=m  TranslationThetaOffset=0  TranslationThetaOffsetUnits=deg  RotationMethod=ArbitraryAxis  RotationAngleUnits=rad  RotationStandardAxis=+Z  RotationAngle=standParams.RigidTransform(193).angle  RotationArbitraryAxis=standParams.RigidTransform(193).axis  FollAlignAxisA=+X  BaseAlignAxisA=+Y  FollAlignAxisB=+Y  BaseAlignAxisB=+Z  RotationSequenceAxes=FollowerAxes  RotationSequence=XYX  RotationSequenceAngles=[0 0 0]  RotationSequenceAnglesUnits=deg  RotationMatrix=[1 0 0; 0 1 0; 0 0 1]
  G : PMIOPort  Side=Left
  connections:
  Solid/RConn1 -- ReferenceFrame/RConn1 -- Transform/RConn1
  Transform/LConn1 -- G/RConn1

== system standModel/Bracket_21_RIGID ==
  ReferenceFrame : sm_lib/Frames and Transforms/Reference Frame
  Solid : sm_lib/Body Elements/File Solid  ExtGeomFileName=Bracket6.step  UnitType=FromFile  ExtGeomFileUnits=m  StepReaderType=HEX  ExportConvexHullGeometry=off  InertiaType=Custom  Mass=standParams.Solid(75).mass  MassUnits=lbm  CenterOfMass=standParams.Solid(75).CoM  CenterOfMassUnits=in  MomentsOfInertia=standParams.Solid(75).MoI  MomentsOfInertiaUnits=lbm*in^2  ProductsOfInertia=standParams.Solid(75).PoI  ProductsOfInertiaUnits=lbm*in^2  BasedOnType=DensityFromFile  Density=1000  DensityUnits=kg/m^3  DoExposeReferenceFrame=on  SerializedFrames=<Frames/>  GraphicType=FromGeometry  MarkerShape=Sphere  MarkerSize=10  GraphicVisPropType=SimpleVisualProperties  GraphicDiffuseColor=standParams.Solid(75).color  GraphicSpecularColor=[0.5 0.5 0.5 1.0]  GraphicAmbientColor=[0.15 0.15 0.15 1.0]  GraphicEmissiveColor=[0.0 0.0 0.0 1.0]  GraphicShininess=75  GraphicOpacity=standParams.Solid(75).opacity
  Transform : sm_lib/Frames and Transforms/Rigid Transform  TranslationMethod=Cartesian  TranslationStandardOffset=0  TranslationLengthUnit=in  TranslationStandardAxis=+Z  TranslationCartesianOffset=standParams.RigidTransform(21).translation  TranslationROffset=0  TranslationROffsetUnits=m  TranslationZOffset=0  TranslationZOffsetUnits=m  TranslationThetaOffset=0  TranslationThetaOffsetUnits=deg  RotationMethod=ArbitraryAxis  RotationAngleUnits=rad  RotationStandardAxis=+Z  RotationAngle=standParams.RigidTransform(21).angle  RotationArbitraryAxis=standParams.RigidTransform(21).axis  FollAlignAxisA=+X  BaseAlignAxisA=+Y  FollAlignAxisB=+Y  BaseAlignAxisB=+Z  RotationSequenceAxes=FollowerAxes  RotationSequence=XYX  RotationSequenceAngles=[0 0 0]  RotationSequenceAnglesUnits=deg  RotationMatrix=[1 0 0; 0 1 0; 0 0 1]
  G : PMIOPort  Side=Left
  connections:
  Solid/RConn1 -- ReferenceFrame/RConn1 -- Transform/RConn1
  Transform/LConn1 -- G/RConn1

== system standModel/Frame_Part_5_RIGID ==
  ReferenceFrame : sm_lib/Frames and Transforms/Reference Frame
  Solid : sm_lib/Body Elements/File Solid  ExtGeomFileName=Frame Part.step  UnitType=FromFile  ExtGeomFileUnits=m  StepReaderType=HEX  ExportConvexHullGeometry=off  InertiaType=Custom  Mass=standParams.Solid(204).mass  MassUnits=lbm  CenterOfMass=standParams.Solid(204).CoM  CenterOfMassUnits=in  MomentsOfInertia=standParams.Solid(204).MoI  MomentsOfInertiaUnits=lbm*in^2  ProductsOfInertia=standParams.Solid(204).PoI  ProductsOfInertiaUnits=lbm*in^2  BasedOnType=DensityFromFile  Density=1000  DensityUnits=kg/m^3  DoExposeReferenceFrame=on  SerializedFrames=<Frames/>  GraphicType=FromGeometry  MarkerShape=Sphere  MarkerSize=10  GraphicVisPropType=SimpleVisualProperties  GraphicDiffuseColor=standParams.Solid(204).color  GraphicSpecularColor=[0.5 0.5 0.5 1.0]  GraphicAmbientColor=[0.15 0.15 0.15 1.0]  GraphicEmissiveColor=[0.0 0.0 0.0 1.0]  GraphicShininess=75  GraphicOpacity=standParams.Solid(204).opacity
  Transform : sm_lib/Frames and Transforms/Rigid Transform  TranslationMethod=Cartesian  TranslationStandardOffset=0  TranslationLengthUnit=in  TranslationStandardAxis=+Z  TranslationCartesianOffset=standParams.RigidTransform(16).translation  TranslationROffset=0  TranslationROffsetUnits=m  TranslationZOffset=0  TranslationZOffsetUnits=m  TranslationThetaOffset=0  TranslationThetaOffsetUnits=deg  RotationMethod=ArbitraryAxis  RotationAngleUnits=rad  RotationStandardAxis=+Z  RotationAngle=standParams.RigidTransform(16).angle  RotationArbitraryAxis=standParams.RigidTransform(16).axis  FollAlignAxisA=+X  BaseAlignAxisA=+Y  FollAlignAxisB=+Y  BaseAlignAxisB=+Z  RotationSequenceAxes=FollowerAxes  RotationSequence=XYX  RotationSequenceAngles=[0 0 0]  RotationSequenceAnglesUnits=deg  RotationMatrix=[1 0 0; 0 1 0; 0 0 1]
  G : PMIOPort  Side=Left
  connections:
  Solid/RConn1 -- ReferenceFrame/RConn1 -- Transform/RConn1
  Transform/LConn1 -- G/RConn1

== system standModel/Frame_Part_6_RIGID ==
  ReferenceFrame : sm_lib/Frames and Transforms/Reference Frame
  Solid : sm_lib/Body Elements/File Solid  ExtGeomFileName=Frame Part1.step  UnitType=FromFile  ExtGeomFileUnits=m  StepReaderType=HEX  ExportConvexHullGeometry=off  InertiaType=Custom  Mass=standParams.Solid(86).mass  MassUnits=lbm  CenterOfMass=standParams.Solid(86).CoM  CenterOfMassUnits=in  MomentsOfInertia=standParams.Solid(86).MoI  MomentsOfInertiaUnits=lbm*in^2  ProductsOfInertia=standParams.Solid(86).PoI  ProductsOfInertiaUnits=lbm*in^2  BasedOnType=DensityFromFile  Density=1000  DensityUnits=kg/m^3  DoExposeReferenceFrame=on  SerializedFrames=<Frames/>  GraphicType=FromGeometry  MarkerShape=Sphere  MarkerSize=10  GraphicVisPropType=SimpleVisualProperties  GraphicDiffuseColor=standParams.Solid(86).color  GraphicSpecularColor=[0.5 0.5 0.5 1.0]  GraphicAmbientColor=[0.15 0.15 0.15 1.0]  GraphicEmissiveColor=[0.0 0.0 0.0 1.0]  GraphicShininess=75  GraphicOpacity=standParams.Solid(86).opacity
  Transform : sm_lib/Frames and Transforms/Rigid Transform  TranslationMethod=Cartesian  TranslationStandardOffset=0  TranslationLengthUnit=in  TranslationStandardAxis=+Z  TranslationCartesianOffset=standParams.RigidTransform(8).translation  TranslationROffset=0  TranslationROffsetUnits=m  TranslationZOffset=0  TranslationZOffsetUnits=m  TranslationThetaOffset=0  TranslationThetaOffsetUnits=deg  RotationMethod=ArbitraryAxis  RotationAngleUnits=rad  RotationStandardAxis=+Z  RotationAngle=standParams.RigidTransform(8).angle  RotationArbitraryAxis=standParams.RigidTransform(8).axis  FollAlignAxisA=+X  BaseAlignAxisA=+Y  FollAlignAxisB=+Y  BaseAlignAxisB=+Z  RotationSequenceAxes=FollowerAxes  RotationSequence=XYX  RotationSequenceAngles=[0 0 0]  RotationSequenceAnglesUnits=deg  RotationMatrix=[1 0 0; 0 1 0; 0 0 1]
  G : PMIOPort  Side=Left
  connections:
  Solid/RConn1 -- ReferenceFrame/RConn1 -- Transform/RConn1
  Transform/LConn1 -- G/RConn1

== system standModel/Hinge_10_RIGID ==
  ReferenceFrame : sm_lib/Frames and Transforms/Reference Frame
  Solid : sm_lib/Body Elements/File Solid  ExtGeomFileName=Hinge.step  UnitType=FromFile  ExtGeomFileUnits=m  StepReaderType=HEX  ExportConvexHullGeometry=off  InertiaType=Custom  Mass=standParams.Solid(31).mass  MassUnits=lbm  CenterOfMass=standParams.Solid(31).CoM  CenterOfMassUnits=in  MomentsOfInertia=standParams.Solid(31).MoI  MomentsOfInertiaUnits=lbm*in^2  ProductsOfInertia=standParams.Solid(31).PoI  ProductsOfInertiaUnits=lbm*in^2  BasedOnType=DensityFromFile  Density=1000  DensityUnits=kg/m^3  DoExposeReferenceFrame=on  SerializedFrames=<Frames/>  GraphicType=FromGeometry  MarkerShape=Sphere  MarkerSize=10  GraphicVisPropType=SimpleVisualProperties  GraphicDiffuseColor=standParams.Solid(31).color  GraphicSpecularColor=[0.5 0.5 0.5 1.0]  GraphicAmbientColor=[0.15 0.15 0.15 1.0]  GraphicEmissiveColor=[0.0 0.0 0.0 1.0]  GraphicShininess=75  GraphicOpacity=standParams.Solid(31).opacity
  Transform : sm_lib/Frames and Transforms/Rigid Transform  TranslationMethod=Cartesian  TranslationStandardOffset=0  TranslationLengthUnit=in  TranslationStandardAxis=+Z  TranslationCartesianOffset=standParams.RigidTransform(63).translation  TranslationROffset=0  TranslationROffsetUnits=m  TranslationZOffset=0  TranslationZOffsetUnits=m  TranslationThetaOffset=0  TranslationThetaOffsetUnits=deg  RotationMethod=ArbitraryAxis  RotationAngleUnits=rad  RotationStandardAxis=+Z  RotationAngle=standParams.RigidTransform(63).angle  RotationArbitraryAxis=standParams.RigidTransform(63).axis  FollAlignAxisA=+X  BaseAlignAxisA=+Y  FollAlignAxisB=+Y  BaseAlignAxisB=+Z  RotationSequenceAxes=FollowerAxes  RotationSequence=XYX  RotationSequenceAngles=[0 0 0]  RotationSequenceAnglesUnits=deg  RotationMatrix=[1 0 0; 0 1 0; 0 0 1]
  G : PMIOPort  Side=Left
  connections:
  Solid/RConn1 -- ReferenceFrame/RConn1 -- Transform/RConn1
  Transform/LConn1 -- G/RConn1

== system standModel/Hinge_11_RIGID ==
  ReferenceFrame : sm_lib/Frames and Transforms/Reference Frame
  Solid : sm_lib/Body Elements/File Solid  ExtGeomFileName=Hinge1.step  UnitType=FromFile  ExtGeomFileUnits=m  StepReaderType=HEX  ExportConvexHullGeometry=off  InertiaType=Custom  Mass=standParams.Solid(167).mass  MassUnits=lbm  CenterOfMass=standParams.Solid(167).CoM  CenterOfMassUnits=in  MomentsOfInertia=standParams.Solid(167).MoI  MomentsOfInertiaUnits=lbm*in^2  ProductsOfInertia=standParams.Solid(167).PoI  ProductsOfInertiaUnits=lbm*in^2  BasedOnType=DensityFromFile  Density=1000  DensityUnits=kg/m^3  DoExposeReferenceFrame=on  SerializedFrames=<Frames/>  GraphicType=FromGeometry  MarkerShape=Sphere  MarkerSize=10  GraphicVisPropType=SimpleVisualProperties  GraphicDiffuseColor=standParams.Solid(167).color  GraphicSpecularColor=[0.5 0.5 0.5 1.0]  GraphicAmbientColor=[0.15 0.15 0.15 1.0]  GraphicEmissiveColor=[0.0 0.0 0.0 1.0]  GraphicShininess=75  GraphicOpacity=standParams.Solid(167).opacity
  Transform : sm_lib/Frames and Transforms/Rigid Transform  TranslationMethod=Cartesian  TranslationStandardOffset=0  TranslationLengthUnit=in  TranslationStandardAxis=+Z  TranslationCartesianOffset=standParams.RigidTransform(27).translation  TranslationROffset=0  TranslationROffsetUnits=m  TranslationZOffset=0  TranslationZOffsetUnits=m  TranslationThetaOffset=0  TranslationThetaOffsetUnits=deg  RotationMethod=ArbitraryAxis  RotationAngleUnits=rad  RotationStandardAxis=+Z  RotationAngle=standParams.RigidTransform(27).angle  RotationArbitraryAxis=standParams.RigidTransform(27).axis  FollAlignAxisA=+X  BaseAlignAxisA=+Y  FollAlignAxisB=+Y  BaseAlignAxisB=+Z  RotationSequenceAxes=FollowerAxes  RotationSequence=XYX  RotationSequenceAngles=[0 0 0]  RotationSequenceAnglesUnits=deg  RotationMatrix=[1 0 0; 0 1 0; 0 0 1]
  G : PMIOPort  Side=Left
  connections:
  Solid/RConn1 -- ReferenceFrame/RConn1 -- Transform/RConn1
  Transform/LConn1 -- G/RConn1

== system standModel/Lock_tabs_13_RIGID ==
  ReferenceFrame : sm_lib/Frames and Transforms/Reference Frame
  Solid : sm_lib/Body Elements/File Solid  ExtGeomFileName=Lock tabs.step  UnitType=FromFile  ExtGeomFileUnits=m  StepReaderType=HEX  ExportConvexHullGeometry=off  InertiaType=Custom  Mass=standParams.Solid(72).mass  MassUnits=lbm  CenterOfMass=standParams.Solid(72).CoM  CenterOfMassUnits=in  MomentsOfInertia=standParams.Solid(72).MoI  MomentsOfInertiaUnits=lbm*in^2  ProductsOfInertia=standParams.Solid(72).PoI  ProductsOfInertiaUnits=lbm*in^2  BasedOnType=DensityFromFile  Density=1000  DensityUnits=kg/m^3  DoExposeReferenceFrame=on  SerializedFrames=<Frames/>  GraphicType=FromGeometry  MarkerShape=Sphere  MarkerSize=10  GraphicVisPropType=SimpleVisualProperties  GraphicDiffuseColor=standParams.Solid(72).color  GraphicSpecularColor=[0.5 0.5 0.5 1.0]  GraphicAmbientColor=[0.15 0.15 0.15 1.0]  GraphicEmissiveColor=[0.0 0.0 0.0 1.0]  GraphicShininess=75  GraphicOpacity=standParams.Solid(72).opacity
  Transform : sm_lib/Frames and Transforms/Rigid Transform  TranslationMethod=Cartesian  TranslationStandardOffset=0  TranslationLengthUnit=in  TranslationStandardAxis=+Z  TranslationCartesianOffset=standParams.RigidTransform(5).translation  TranslationROffset=0  TranslationROffsetUnits=m  TranslationZOffset=0  TranslationZOffsetUnits=m  TranslationThetaOffset=0  TranslationThetaOffsetUnits=deg  RotationMethod=ArbitraryAxis  RotationAngleUnits=rad  RotationStandardAxis=+Z  RotationAngle=standParams.RigidTransform(5).angle  RotationArbitraryAxis=standParams.RigidTransform(5).axis  FollAlignAxisA=+X  BaseAlignAxisA=+Y  FollAlignAxisB=+Y  BaseAlignAxisB=+Z  RotationSequenceAxes=FollowerAxes  RotationSequence=XYX  RotationSequenceAngles=[0 0 0]  RotationSequenceAnglesUnits=deg  RotationMatrix=[1 0 0; 0 1 0; 0 0 1]
  G : PMIOPort  Side=Left
  connections:
  Solid/RConn1 -- ReferenceFrame/RConn1 -- Transform/RConn1
  Transform/LConn1 -- G/RConn1
